simulink model "crash_original"  (R2021b)
settings: Solver=FixedStepAuto  StartTime=0.0  StopTime=10.0  RelTol=1e-3
undefined symbols (not defined in the file): DiscIntNeverNeededParam, sigbuilder_block
libraries: simulink x292, slpidlib x133
(part 1 of 12)
settings Model: Creator=cyfuzz  LastModifiedBy=cemery
settings SolverCC: AlgebraicLoopSolver=TrustRegion
settings DataIOCC: ReturnWorkspaceOutputs=off
settings DebuggingCC: SFMachineParentedDataDiag=warning  ArithmeticOperatorsInVariantConditions=warning
settings SFSimCC: SimUseLocalCustomCode=off  CustomCodeUndefinedFunction=UseInterfaceOnly
settings RTWCC: RTWUseLocalCustomCode=off
settings CodeAppCC: StateflowObjectComments=on

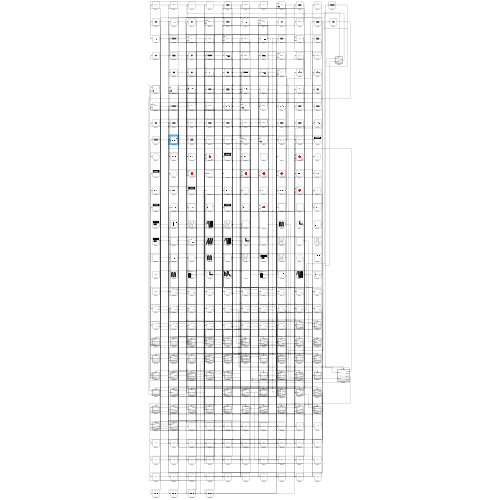
[thumbnail: Simulink's stored preview of the top-level diagram]
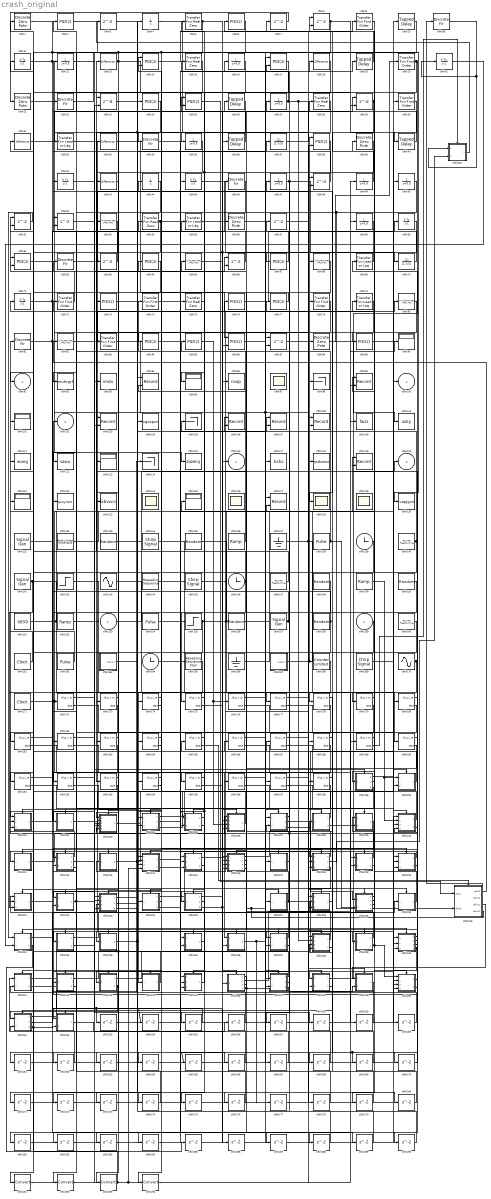
== system crash_original ==
  cfblk153 : Inport
  cfblk159 : Inport  Port=2
  cfblk{1,21,39,56,88} (5 alike) : DiscreteZeroPole  Poles=[0 0.5]  Gain=1
  cfblk{10,19,26,36,40} (5 alike) : simulink/Discrete/Tapped Delay  vinit=0.0  samptime=-1  NumDelays=1  DelayOrder=Oldest  includeCurrent=off
  cfblk{90,95,101,113,121,125} (6 alike) : Display
  cfblk103 : Record  FileSettingsInternal="{\"entries\":[{\"content\":{\"excelSettings\":{\"content\":{},\"type\":\"Streamout.ExcelSettings\"}},\"type\":\"Streamout.FileSettingStorage\",\"uuid\":\"30172691-4b6d-43b6-90c1-8d96ffbb56b2\"}],\"packageUris\":[\"http://schema.mathworks.com/mf0/streamout_blocks/R2020a\"],\"version\":\"1.0\"}"  Layout=[1 1]  SignalsInternal="{\"entries\":[{\"content\":{\"signals\":[{\"content\":{\"blockPath\":[\"crash_original/cfblk103\"],\"channel\":[],\"dimensions\":[1],\"domain\":\"crash_original/cfblk103\",\"lineColor\":\"#a2142f\",\"plots\":[1],\"port\":1,\"sid\":[],\"signalID\":25354,\"signalName\":\"XY Graph:1\"},\"type\":\"RecordBlkView.Signal\",\"uuid\":\"414546f9-114d-477c-ba68-cfa88be5a9bf\"},{\"content\":{\"blockPath\":[\"crash_original/cfblk103\"],\"channel\":[],\"dimensions\":[1],\"domain\":\"crash_original/cfblk103\",\"lineColor\":\"#139fff\",\"plots\":[1],\"port\":2,\"sid\":[],\"signalID\":25357,\"signalName\":\"XY Graph:2\"},\"type\":\"RecordBlkView.Signal\",\"uuid\":\"96b3544b-9d06-4962-b904-c7b3bf9edbf5\"}]},\"type\":\"RecordBlkView.InputSignals\",\"uuid\":\"c1b797b7-706f-480f-856e-f9fd9aac0f38\"}],\"packageUris\":[\"http://schema.mathworks.com/mf0/streamout_blocks/R2020a\"],\"version\":\"1.0\"}"  VisualizationBindings="{\"xyplotplugin\":{\"info\":[{\"series\":[{\"bindingParametersList\":[{\"parameter\":\"X-Axis\",\"signalID\":25354,\"signalName\":\"XY Graph:1\"},{\"parameter\":\"Y-Axis\",\"signalID\":25357,\"signalName\":\"XY Graph:2\"}],\"seriesID\":52165}],\"subplotID\":1}]}}"  CompatibilityTag=XY  st=-1
  cfblk104 : ToWorkspace  VariableName=cgozpzv  SaveFormat=Timeseries  SampleTime=-1
  cfblk105 : Terminator
  cfblk106 : Record  FileSettingsInternal="{\"entries\":[{\"content\":{\"excelSettings\":{\"content\":{},\"type\":\"Streamout.ExcelSettings\"}},\"type\":\"Streamout.FileSettingStorage\",\"uuid\":\"5105aa24-88b4-4d22-8fbb-db2b517dd038\"}],\"packageUris\":[\"http://schema.mathworks.com/mf0/streamout_blocks/R2020a\"],\"version\":\"1.0\"}"  Layout=[1 1]  SignalsInternal="{\"entries\":[{\"content\":{\"signals\":[{\"content\":{\"blockPath\":[\"crash_original/cfblk106\"],\"channel\":[],\"dimensions\":[1],\"domain\":\"crash_original/cfblk106\",\"lineColor\":\"#a2142f\",\"plots\":[1],\"port\":1,\"sid\":[],\"signalID\":25346,\"signalName\":\"XY Graph:1\"},\"type\":\"RecordBlkView.Signal\",\"uuid\":\"9204552f-2c26-4ac5-bb3a-39315a682c7e\"},{\"content\":{\"blockPath\":[\"crash_original/cfblk106\"],\"channel\":[],\"dimensions\":[1],\"domain\":\"crash_original/cfblk106\",\"lineColor\":\"#139fff\",\"plots\":[1],\"port\":2,\"sid\":[],\"signalID\":25349,\"signalName\":\"XY Graph:2\"},\"type\":\"RecordBlkView.Signal\",\"uuid\":\"12e95a38-9289-47da-aacf-37fae59f2bfe\"}]},\"type\":\"RecordBlkView.InputSignals\",\"uuid\":\"d2112c08-a194-4577-8bfc-846eb5e090f8\"}],\"packageUris\":[\"http://schema.mathworks.com/mf0/streamout_blocks/R2020a\"],\"version\":\"1.0\"}"  VisualizationBindings="{\"xyplotplugin\":{\"info\":[{\"series\":[{\"bindingParametersList\":[{\"parameter\":\"X-Axis\",\"signalID\":25346,\"signalName\":\"XY Graph:1\"},{\"parameter\":\"Y-Axis\",\"signalID\":25349,\"signalName\":\"XY Graph:2\"}],\"seriesID\":14933}],\"subplotID\":1}]}}"  CompatibilityTag=XY  st=-1
  cfblk107 : Record  FileSettingsInternal="{\"entries\":[{\"content\":{\"excelSettings\":{\"content\":{},\"type\":\"Streamout.ExcelSettings\"}},\"type\":\"Streamout.FileSettingStorage\",\"uuid\":\"9a455097-a817-49c6-a5c0-eb2ae5036dd7\"}],\"packageUris\":[\"http://schema.mathworks.com/mf0/streamout_blocks/R2020a\"],\"version\":\"1.0\"}"  Layout=[1 1]  SignalsInternal="{\"entries\":[{\"content\":{\"signals\":[{\"content\":{\"blockPath\":[\"crash_original/cfblk107\"],\"channel\":[],\"dimensions\":[1],\"domain\":\"crash_original/cfblk107\",\"lineColor\":\"#a2142f\",\"plots\":[1],\"port\":1,\"sid\":[],\"signalID\":25338,\"signalName\":\"XY Graph:1\"},\"type\":\"RecordBlkView.Signal\",\"uuid\":\"72b46ba4-58e1-4237-a289-6594da422004\"},{\"content\":{\"blockPath\":[\"crash_original/cfblk107\"],\"channel\":[],\"dimensions\":[1],\"domain\":\"crash_original/cfblk107\",\"lineColor\":\"#139fff\",\"plots\":[1],\"port\":2,\"sid\":[],\"signalID\":25341,\"signalName\":\"XY Graph:2\"},\"type\":\"RecordBlkView.Signal\",\"uuid\":\"e835df7f-5567-4283-ab7a-943fc1d95c97\"}]},\"type\":\"RecordBlkView.InputSignals\",\"uuid\":\"dcc1e580-6fae-4788-903d-9782004bc5fd\"}],\"packageUris\":[\"http://schema.mathworks.com/mf0/streamout_blocks/R2020a\"],\"version\":\"1.0\"}"  VisualizationBindings="{\"xyplotplugin\":{\"info\":[{\"series\":[{\"bindingParametersList\":[{\"parameter\":\"X-Axis\",\"signalID\":25338,\"signalName\":\"XY Graph:1\"},{\"parameter\":\"Y-Axis\",\"signalID\":25341,\"signalName\":\"XY Graph:2\"}],\"seriesID\":31324}],\"subplotID\":1}]}}"  CompatibilityTag=XY  st=-1
  cfblk108 : Record  FileSettingsInternal="{\"entries\":[{\"content\":{\"excelSettings\":{\"content\":{},\"type\":\"Streamout.ExcelSettings\"}},\"type\":\"Streamout.FileSettingStorage\",\"uuid\":\"0bf2bf5e-f4e3-4816-82a7-4f814904066c\"}],\"packageUris\":[\"http://schema.mathworks.com/mf0/streamout_blocks/R2020a\"],\"version\":\"1.0\"}"  Layout=[1 1]  SignalsInternal="{\"entries\":[{\"content\":{\"signals\":[{\"content\":{\"blockPath\":[\"crash_original/cfblk108\"],\"channel\":[],\"dimensions\":[1],\"domain\":\"crash_original/cfblk108\",\"lineColor\":\"#a2142f\",\"plots\":[1],\"port\":1,\"sid\":[],\"signalID\":25330,\"signalName\":\"XY Graph:1\"},\"type\":\"RecordBlkView.Signal\",\"uuid\":\"ec0f48f3-9d1b-4216-bb21-ef0bcc557efa\"},{\"content\":{\"blockPath\":[\"crash_original/cfblk108\"],\"channel\":[],\"dimensions\":[1],\"domain\":\"crash_original/cfblk108\",\"lineColor\":\"#139fff\",\"plots\":[1],\"port\":2,\"sid\":[],\"signalID\":25333,\"signalName\":\"XY Graph:2\"},\"type\":\"RecordBlkView.Signal\",\"uuid\":\"97f765a4-0795-4aab-bdad-c330e4c16f83\"}]},\"type\":\"RecordBlkView.InputSignals\",\"uuid\":\"3c2073ef-6d47-42f6-9099-379ba4442adb\"}],\"packageUris\":[\"http://schema.mathworks.com/mf0/streamout_blocks/R2020a\"],\"version\":\"1.0\"}"  VisualizationBindings="{\"xyplotplugin\":{\"info\":[{\"series\":[{\"bindingParametersList\":[{\"parameter\":\"X-Axis\",\"signalID\":25330,\"signalName\":\"XY Graph:1\"},{\"parameter\":\"Y-Axis\",\"signalID\":25333,\"signalName\":\"XY Graph:2\"}],\"seriesID\":8656}],\"subplotID\":1}]}}"  CompatibilityTag=XY  st=-1
  cfblk109 : ToFile  Filename=fwzz  SaveFormat=Timeseries
  cfblk{11,41..42,45,60,71} (6 alike) : DiscreteIntegrator  ICPrevOutput=DiscIntNeverNeededParam  ICPrevScaledInput=DiscIntNeverNeededParam
  cfblk110 : ToFile  Filename=azky  SaveFormat=Timeseries
  cfblk111 : ToFile  Filename=wang  SaveFormat=Timeseries
  cfblk112 : ToFile  Filename=sawu  SaveFormat=Timeseries
  cfblk114 : Terminator
  cfblk115 : ToWorkspace  VariableName=zazenij  SaveFormat=Timeseries  SampleTime=-1
  cfblk117 : ToFile  Filename=bshz  SaveFormat=Timeseries
  cfblk118 : ToWorkspace  VariableName=rpdzwsv  SaveFormat=Timeseries  SampleTime=-1
  cfblk119 : Record  FileSettingsInternal="{\"entries\":[{\"content\":{\"excelSettings\":{\"content\":{},\"type\":\"Streamout.ExcelSettings\"}},\"type\":\"Streamout.FileSettingStorage\",\"uuid\":\"fee27d59-1ddc-47f4-9b88-6ce813c8d426\"}],\"packageUris\":[\"http://schema.mathworks.com/mf0/streamout_blocks/R2020a\"],\"version\":\"1.0\"}"  Layout=[1 1]  SignalsInternal="{\"entries\":[{\"content\":{\"signals\":[{\"content\":{\"blockPath\":[\"crash_original/cfblk119\"],\"channel\":[],\"dimensions\":[1],\"domain\":\"crash_original/cfblk119\",\"lineColor\":\"#a2142f\",\"plots\":[1],\"port\":1,\"sid\":[],\"signalID\":25322,\"signalName\":\"XY Graph:1\"},\"type\":\"RecordBlkView.Signal\",\"uuid\":\"effbb9bf-c420-46b1-a7d1-1e032b18154d\"},{\"content\":{\"blockPath\":[\"crash_original/cfblk119\"],\"channel\":[],\"dimensions\":[1],\"domain\":\"crash_original/cfblk119\",\"lineColor\":\"#139fff\",\"plots\":[1],\"port\":2,\"sid\":[],\"signalID\":25325,\"signalName\":\"XY Graph:2\"},\"type\":\"RecordBlkView.Signal\",\"uuid\":\"bb2f82c4-e824-49d1-9fc8-a47dada03492\"}]},\"type\":\"RecordBlkView.InputSignals\",\"uuid\":\"82b3e0f0-e2fd-4ae7-a1eb-90a31382d85a\"}],\"packageUris\":[\"http://schema.mathworks.com/mf0/streamout_blocks/R2020a\"],\"version\":\"1.0\"}"  VisualizationBindings="{\"xyplotplugin\":{\"info\":[{\"series\":[{\"bindingParametersList\":[{\"parameter\":\"X-Axis\",\"signalID\":25322,\"signalName\":\"XY Graph:1\"},{\"parameter\":\"Y-Axis\",\"signalID\":25325,\"signalName\":\"XY Graph:2\"}],\"seriesID\":29524}],\"subplotID\":1}]}}"  CompatibilityTag=XY  st=-1
  cfblk{12,16,27,35,47,49..50,59} (8 alike) : DiscreteTransferFcn  SampleTime=1
  cfblk122 : ToWorkspace  VariableName=qvnyrom  SaveFormat=Timeseries  SampleTime=-1
  cfblk123 : ToWorkspace  VariableName=lxbvxco  SaveFormat=Timeseries  SampleTime=-1
  cfblk{97,124,126,128..129} (5 alike) : Scope
      cfblk124 settings: Floating=on
      cfblk126 settings: Floating=on
      cfblk129 settings: Floating=on
      cfblk97 settings: Floating=on
  cfblk127 : Record  FileSettingsInternal="{\"entries\":[{\"content\":{\"excelSettings\":{\"content\":{},\"type\":\"Streamout.ExcelSettings\"}},\"type\":\"Streamout.FileSettingStorage\",\"uuid\":\"83428cd0-c40d-4b56-9453-87c774a237f4\"}],\"packageUris\":[\"http://schema.mathworks.com/mf0/streamout_blocks/R2020a\"],\"version\":\"1.0\"}"  Layout=[1 1]  SignalsInternal="{\"entries\":[{\"content\":{\"signals\":[{\"content\":{\"blockPath\":[\"crash_original/cfblk127\"],\"channel\":[],\"dimensions\":[1],\"domain\":\"crash_original/cfblk127\",\"lineColor\":\"#a2142f\",\"plots\":[1],\"port\":1,\"sid\":[],\"signalID\":25314,\"signalName\":\"XY Graph:1\"},\"type\":\"RecordBlkView.Signal\",\"uuid\":\"4ffe00b0-219f-48e9-9eae-af36f4ef0fcf\"},{\"content\":{\"blockPath\":[\"crash_original/cfblk127\"],\"channel\":[],\"dimensions\":[1],\"domain\":\"crash_original/cfblk127\",\"lineColor\":\"#139fff\",\"plots\":[1],\"port\":2,\"sid\":[],\"signalID\":25317,\"signalName\":\"XY Graph:2\"},\"type\":\"RecordBlkView.Signal\",\"uuid\":\"f85c7929-cc6b-466a-b10c-b0d057f1a651\"}]},\"type\":\"RecordBlkView.InputSignals\",\"uuid\":\"7a008c7c-a3ea-4e7c-8ad4-a9eac3daa760\"}],\"packageUris\":[\"http://schema.mathworks.com/mf0/streamout_blocks/R2020a\"],\"version\":\"1.0\"}"  VisualizationBindings="{\"xyplotplugin\":{\"info\":[{\"series\":[{\"bindingParametersList\":[{\"parameter\":\"X-Axis\",\"signalID\":25314,\"signalName\":\"XY Graph:1\"},{\"parameter\":\"Y-Axis\",\"signalID\":25317,\"signalName\":\"XY Graph:2\"}],\"seriesID\":431}],\"subplotID\":1}]}}"  CompatibilityTag=XY  st=-1
  cfblk{13,18,31,33,43} (5 alike) : simulink/Discrete/Difference  ICPrevInput=0.0  OutMin=[]  OutMax=[]  OutDataTypeStr=Inherit: Inherit via back propagation  OutDataType=fixdt(1, 16)  OutScaling=2^-10  DoSatur=off
  cfblk130 : ToWorkspace  VariableName=vapjgvn  SaveFormat=Timeseries  SampleTime=-1
  cfblk131 : SignalGenerator  Units=rad/sec
  cfblk132 : simulink/Sources/Band-Limited White Noise  Cov=[0.1]  Ts=0.1  seed=[23341]
  cfblk{133,135,148,156,158} (5 alike) : UniformRandomNumber  SampleTime=0.1
  cfblk134 : simulink/Sources/Chirp Signal  f1=0.1  T=100  f2=1
  cfblk136 : simulink/Sources/Ramp  slope=1  start=0  InitialOutput=0
  cfblk137 : Ground
  cfblk138 : DiscretePulseGenerator  PulseType=Time based  Period=10  PulseWidth=5
  cfblk139 : Clock
  cfblk{14,17,25,38,61,86} (6 alike) : slpidlib/PID Controller (2DOF)  Controller=PID  Form=Parallel  TimeDomain=Discrete-time  UseExternalTs=off  SampleTime=1  IntegratorMethod=Forward Euler  FilterMethod=Forward Euler  ControllerParametersSource=internal  P=1  I=1  D=0  UseFilter=on  N=100  b=1  c=1  TunerSelectOption=Transfer Function Based (PID Tuner App)  InitialConditionSource=internal  InitialConditionForIntegrator=0  InitialConditionForFilter=0  DifferentiatorICPrevScaledInput=0  ExternalReset=none  TrackingMode=off  Kt=1  LimitOutput=off  SatLimitsSource=internal  UpperSaturationLimit=inf  LowerSaturationLimit=-inf  LinearizeAsGain=off  AntiWindupMode=none  Kb=1  POutMin=[]  POutMax=[]  IOutMin=[]  IOutMax=[]  DOutMin=[]  DOutMax=[]  NOutMin=[]  NOutMax=[]  bOutMin=[]  bOutMax=[]  cOutMin=[]  cOutMax=[]  SumOutMin=[]  SumOutMax=[]  SaturationOutMin=[]  SaturationOutMax=[]  PParamMin=[]  PParamMax=[]  IParamMin=[]  IParamMax=[]  DParamMin=[]  DParamMax=[]  NParamMin=[]  NParamMax=[]  bParamMin=[]  bParamMax=[]  cParamMin=[]  cParamMax=[]  KbParamMin=[]  KbParamMax=[]  KtParamMin=[]  KtParamMax=[]  KbOutMin=[]  KbOutMax=[]  KtOutMin=[]  KtOutMax=[]  IntegratorOutMin=[]  IntegratorOutMax=[]  FilterOutMin=[]  FilterOutMax=[]  SumI1OutMin=[]  SumI1OutMax=[]  SumI2OutMin=[]  SumI2OutMax=[]  SumI3OutMin=[]  SumI3OutMax=[]  SumI4OutMin=[]  SumI4OutMax=[]  SumDOutMin=[]  SumDOutMax=[]  Sum1OutMin=[]  Sum1OutMax=[]  Sum2OutMin=[]  Sum2OutMax=[]  Sum3OutMin=[]  Sum3OutMax=[]  DifferentiatorOutMin=[]  DifferentiatorOutMax=[]  FilterDiffOutCoefMin=[]  FilterDiffOutCoefMax=[]  ReciprocalOutMin=[]  ReciprocalOutMax=[]  SumDenOutMin=[]  SumDenOutMax=[]  SumNumOutMin=[]  SumNumOutMax=[]  DivideOutMin=[]  DivideOutMax=[]  UdiffTsProdOutMin=[]  UdiffTsProdOutMax=[]  NTsProdOutMin=[]  NTsProdOutMax=[]  UintegralTsProdOutMin=[]  UintegralTsProdOutMax=[]  UngainTsProdOutMin=[]  UngainTsProdOutMax=[]  IntegratorContinuousStateAttributes=''  IntegratorStateMustResolveToSignalObject=off  IntegratorRTWStateStorageClass=Auto  FilterContinuousStateAttributes=''  FilterStateMustResolveToSignalObject=off  FilterRTWStateStorageClass=Auto  ParallelPVariant=InternalParameters  IdealPVariant=Disabled  IVariant=InternalParameters  DVariant=InternalParameters  bVariant=InternalParameters  cVariant=InternalParameters  IntegratorVariant=Discrete  SatVariant=Disabled  AWVariant=Passthrough  PCopyVariant=Disabled  TRVariant=Disabled  FdbkBlocksVariant=Forward  IdealPFdbkVariant=Disabled  SatFdbkVariant=Disabled  DerivativeFilterVariant=ForwardEulerFilter  NVariant=InternalParameters  NCopyVariant=Disabled  FilterICVariant=InternalICsFilter  IntegratorICVariant=InternalICs  ExternalResetVariant=Disabled  TRSumVariant=Passthrough  SumFdbkVariant=Disabled  SumVariant=Sum_PID  TsampFilterVariant=InternalTs  TsampNgainVariant=Passthrough  TsampIntegralVariant=Passthrough  ExternalSaturationOutDataTypeStr=Inherit: Same as second input
      settings: SourceProductBaseCode=SL
  cfblk140 : simulink/Sources/Counter Free-Running  NumBits=16  tsamp=-1
  cfblk141 : SignalGenerator  Units=rad/sec
  cfblk142 : Step  After=57  SampleTime=0
  cfblk143 : Sin  SampleTime=0
  cfblk144 : simulink/Sources/Repeating Sequence  rep_seq_t=[0 2]  rep_seq_y=[0 2]
  cfblk145 : simulink/Sources/Chirp Signal  f1=0.1  T=100  f2=1
  cfblk146 : Clock
  cfblk147 : simulink/Sources/Counter Free-Running  NumBits=16  tsamp=-1
  cfblk149 : simulink/Sources/Ramp  slope=1  start=0  InitialOutput=0
  cfblk{5,15,28,54,75} (5 alike) : simulink/Discrete/Transfer Fcn Real Zero  ZeroZ=0.75  ICPrevInput=0.0  DoSatur=off
      settings: SourceProductBaseCode=SL
  cfblk150 : RandomNumber  SampleTime=0.1
  cfblk151 : Constant  Value=9859
  cfblk152 : simulink/Sources/Ramp  slope=1  start=0  InitialOutput=0
  cfblk154 : DiscretePulseGenerator  PulseType=Time based  Period=10  PulseWidth=5
  cfblk155 : Step  After=75  SampleTime=0
  cfblk157 : SignalGenerator  Units=rad/sec
  cfblk160 : simulink/Sources/Counter Free-Running  NumBits=16  tsamp=-1
  cfblk161 : DigitalClock
  cfblk162 : DiscretePulseGenerator  PulseType=Time based  Period=10  PulseWidth=5
  cfblk163 : Subsystem  Tag=STV Subsys  LoadFcn=sigbuilder_block('load');  StartFcn=sigbuilder_block('start');  StopFcn=sigbuilder_block('stop');  ClipboardFcn=sigbuilder_block('clipboard');  mask(Sigbuilder block){tuvar=[0:10]}
      mask help: Simulink:masks:SigbuilderBlock_MD
      mask init:
      | if ~strcmp(get_param(bdroot(gcbh),'SimulationStatus'),'stopped') tuvar = sigbuilder_block('maskInit'); end
      settings: CopyFcn=sigbuilder_block('copy');  DeleteFcn=sigbuilder_block('delete');  ModelCloseFcn=sigbuilder_block('modelClose');  PreSaveFcn=sigbuilder_block('preSave');  PauseFcn=sigbuilder_block('pause');  ContinueFcn=sigbuilder_block('continue');  NameChangeFcn=sigbuilder_block('namechange');  OpenFcn=sigbuilder_block('open',[437.6 199.2 550.4 400 ]);  CloseFcn=sigbuilder_block('close');
      mask Display: plot(0, 0, 100, 100,[2, 2, 32, 32, 2], [68, 8, 8, 68, 68],[32, 2], [38, 38], [32, 19, 2],[53, 60, 44], [32, 17, 17, 2],[16, 16, 31, 31]);txt = getActiveGroup(gcbh);text(2, 100, txt,'verticalAlignment', 'top');
  cfblk164 : Clock
  cfblk165 : simulink/Sources/Repeating Sequence Stair  OutValues=[3 1 4 2 1].'  tsamp=-1  OutMin=[]  OutMax=[]  OutDataTypeStr=double  OutputDataTypeScalingMode=double  OutDataType=fixdt(0,8)  ConRadixGroup=Best Precision: Vector-wise  OutScaling=2^-12
  cfblk166 : Ground
  cfblk167 : Subsystem  Tag=STV Subsys  LoadFcn=sigbuilder_block('load');  StartFcn=sigbuilder_block('start');  StopFcn=sigbuilder_block('stop');  ClipboardFcn=sigbuilder_block('clipboard');  mask(Sigbuilder block){tuvar=[0:10]}
      mask help: Simulink:masks:SigbuilderBlock_MD
      mask init:
      | if ~strcmp(get_param(bdroot(gcbh),'SimulationStatus'),'stopped') tuvar = sigbuilder_block('maskInit'); end
      settings: CopyFcn=sigbuilder_block('copy');  DeleteFcn=sigbuilder_block('delete');  ModelCloseFcn=sigbuilder_block('modelClose');  PreSaveFcn=sigbuilder_block('preSave');  PauseFcn=sigbuilder_block('pause');  ContinueFcn=sigbuilder_block('continue');  NameChangeFcn=sigbuilder_block('namechange');  OpenFcn=sigbuilder_block('open',[437.6 199.2 550.4 400 ]);  CloseFcn=sigbuilder_block('close');
      mask Display: plot(0, 0, 100, 100,[2, 2, 32, 32, 2], [68, 8, 8, 68, 68],[32, 2], [38, 38], [32, 19, 2],[53, 60, 44], [32, 17, 17, 2],[16, 16, 31, 31]);txt = getActiveGroup(gcbh);text(2, 100, txt,'verticalAlignment', 'top');
  cfblk168 : simulink/Sources/Counter Limited  uplimit=7  tsamp=-1
  cfblk169 : simulink/Sources/Chirp Signal  f1=0.1  T=100  f2=1
  cfblk170 : Sin  SampleTime=0
  cfblk171 : DigitalClock
  cfblk{172..198} (27 alike) : If  SampleTime=1
  cfblk199 : Subsystem  TreatAsAtomicUnit=on
  cfblk{2,6,24,64,67,73,76..77,84..85,89} (11 alike) : slpidlib/PID Controller  Controller=PID  Form=Parallel  TimeDomain=Discrete-time  UseExternalTs=off  SampleTime=1  IntegratorMethod=Forward Euler  FilterMethod=Forward Euler  ControllerParametersSource=internal  P=1  I=1  D=0  UseFilter=on  N=100  TunerSelectOption=Transfer Function Based (PID Tuner App)  InitialConditionSource=internal  InitialConditionForIntegrator=0  InitialConditionForFilter=0  DifferentiatorICPrevScaledInput=0  ExternalReset=none  TrackingMode=off  Kt=1  LimitOutput=off  SatLimitsSource=internal  UpperSaturationLimit=inf  LowerSaturationLimit=-inf  LinearizeAsGain=off  AntiWindupMode=none  Kb=1  POutMin=[]  POutMax=[]  IOutMin=[]  IOutMax=[]  DOutMin=[]  DOutMax=[]  NOutMin=[]  NOutMax=[]  SumOutMin=[]  SumOutMax=[]  SaturationOutMin=[]  SaturationOutMax=[]  PParamMin=[]  PParamMax=[]  IParamMin=[]  IParamMax=[]  DParamMin=[]  DParamMax=[]  NParamMin=[]  NParamMax=[]  KbParamMin=[]  KbParamMax=[]  KtParamMin=[]  KtParamMax=[]  KbOutMin=[]  KbOutMax=[]  KtOutMin=[]  KtOutMax=[]  IntegratorOutMin=[]  IntegratorOutMax=[]  FilterOutMin=[]  FilterOutMax=[]  SumI1OutMin=[]  SumI1OutMax=[]  SumI2OutMin=[]  SumI2OutMax=[]  SumI3OutMin=[]  SumI3OutMax=[]  SumI4OutMin=[]  SumI4OutMax=[]  SumDOutMin=[]  SumDOutMax=[]  DifferentiatorOutMin=[]  DifferentiatorOutMax=[]  FilterDiffOutCoefMin=[]  FilterDiffOutCoefMax=[]  ReciprocalOutMin=[]  ReciprocalOutMax=[]  SumDenOutMin=[]  SumDenOutMax=[]  SumNumOutMin=[]  SumNumOutMax=[]  DivideOutMin=[]  DivideOutMax=[]  UdiffTsProdOutMin=[]  UdiffTsProdOutMax=[]  NTsProdOutMin=[]  NTsProdOutMax=[]  UintegralTsProdOutMin=[]  UintegralTsProdOutMax=[]  UngainTsProdOutMin=[]  UngainTsProdOutMax=[]  IntegratorContinuousStateAttributes=''  IntegratorStateMustResolveToSignalObject=off  IntegratorRTWStateStorageClass=Auto  FilterContinuousStateAttributes=''  FilterStateMustResolveToSignalObject=off  FilterRTWStateStorageClass=Auto  ParallelPVariant=InternalParameters  IdealPVariant=Disabled  IVariant=InternalParameters  DVariant=InternalParameters  IntegratorVariant=Discrete  SatVariant=Disabled  AWVariant=Passthrough  PCopyVariant=Disabled  TRVariant=Disabled  FdbkBlocksVariant=Forward  IdealPFdbkVariant=Disabled  SatFdbkVariant=Disabled  DerivativeFilterVariant=ForwardEulerFilter  NVariant=InternalParameters  NCopyVariant=Disabled  FilterICVariant=InternalICsFilter  IntegratorICVariant=InternalICs  ExternalResetVariant=Disabled  TRSumVariant=Passthrough  SumFdbkVariant=Disabled  SumVariant=Sum_PID  TsampFilterVariant=InternalTs  TsampNgainVariant=Passthrough  TsampIntegralVariant=Passthrough  ExternalSaturationOutDataTypeStr=Inherit: Same as second input
  cfblk{9,20,30,72,74,78,83} (7 alike) : simulink/Discrete/Transfer Fcn First Order  PoleZ=0.95  ICPrevOutput=0.0  DoSatur=off
  cfblk200 : Subsystem  TreatAsAtomicUnit=on
  cfblk201 : Subsystem  TreatAsAtomicUnit=on
  cfblk202 : Subsystem  TreatAsAtomicUnit=on
  cfblk203 : Subsystem  TreatAsAtomicUnit=on
  cfblk204 : Subsystem  TreatAsAtomicUnit=on
  cfblk205 : Subsystem  TreatAsAtomicUnit=on
  cfblk206 : Subsystem  TreatAsAtomicUnit=on
  cfblk207 : Subsystem  TreatAsAtomicUnit=on
  cfblk208 : Subsystem  TreatAsAtomicUnit=on
  cfblk209 : Subsystem  TreatAsAtomicUnit=on
  cfblk210 : Subsystem  TreatAsAtomicUnit=on
  cfblk211 : Subsystem  TreatAsAtomicUnit=on
  cfblk212 : Subsystem  TreatAsAtomicUnit=on
  cfblk213 : Subsystem  TreatAsAtomicUnit=on
  cfblk214 : Subsystem  TreatAsAtomicUnit=on
  cfblk215 : Subsystem  TreatAsAtomicUnit=on
  cfblk216 : Subsystem  TreatAsAtomicUnit=on
  cfblk217 : Subsystem  TreatAsAtomicUnit=on
  cfblk218 : Subsystem  TreatAsAtomicUnit=on
  cfblk219 : Subsystem  TreatAsAtomicUnit=on
  cfblk{22,34,46,58,62,81} (6 alike) : DiscreteFir  SampleTime=1
  cfblk220 : Subsystem  TreatAsAtomicUnit=on
  cfblk221 : Subsystem  TreatAsAtomicUnit=on
  cfblk222 : Subsystem  TreatAsAtomicUnit=on
  cfblk223 : Subsystem  TreatAsAtomicUnit=on
  cfblk224 : Subsystem  TreatAsAtomicUnit=on
  cfblk225 : Subsystem  TreatAsAtomicUnit=on
  cfblk226 : Subsystem  TreatAsAtomicUnit=on
  cfblk227 : Subsystem  TreatAsAtomicUnit=on
  cfblk228 : Subsystem  TreatAsAtomicUnit=on
  cfblk229 : Subsystem  TreatAsAtomicUnit=on
  cfblk23 : Delay  DelayLengthSource=Input port  SampleTime=1
      settings: InputPortMap=u0,p1
  cfblk230 : Subsystem  TreatAsAtomicUnit=on
  cfblk231 : Subsystem  TreatAsAtomicUnit=on
  cfblk232 : Subsystem  TreatAsAtomicUnit=on
  cfblk233 : Subsystem  TreatAsAtomicUnit=on
  cfblk234 : Subsystem  TreatAsAtomicUnit=on
  cfblk235 : Subsystem  TreatAsAtomicUnit=on
  cfblk236 : Subsystem  TreatAsAtomicUnit=on
  cfblk237 : Subsystem  TreatAsAtomicUnit=on
  cfblk238 : Subsystem  TreatAsAtomicUnit=on
  cfblk239 : Subsystem  TreatAsAtomicUnit=on
  cfblk240 : Subsystem  TreatAsAtomicUnit=on
  cfblk241 : Subsystem  TreatAsAtomicUnit=on
  cfblk242 : Subsystem  TreatAsAtomicUnit=on
  cfblk243 : Subsystem  TreatAsAtomicUnit=on
  cfblk244 : Subsystem  TreatAsAtomicUnit=on
  cfblk245 : Subsystem  TreatAsAtomicUnit=on
  cfblk246 : Subsystem  TreatAsAtomicUnit=on
  cfblk247 : Subsystem  TreatAsAtomicUnit=on
  cfblk248 : Subsystem  TreatAsAtomicUnit=on
  cfblk249 : Subsystem  TreatAsAtomicUnit=on
  cfblk250 : Subsystem  TreatAsAtomicUnit=on
  cfblk251 : Subsystem  TreatAsAtomicUnit=on
  cfblk252 : Subsystem  TreatAsAtomicUnit=on
  cfblk{3,7,57,63,253..290} (42 alike) : Delay  SampleTime=1
  cfblk29 : Delay  DelayLengthSource=Input port  SampleTime=1
      settings: InputPortMap=u0,p1
  cfblk{291..294} (4 alike) : DataTypeConversion
  cfblk{32,55,69,79} (4 alike) : simulink/Discrete/Transfer Fcn Lead or Lag  PoleZ=0.95  ZeroZ=0.75  ICPrevOutput=0.0  ICPrevInput=0.0  DoSatur=off
      settings: SourceProductBaseCode=SL
  cfblk37 : DiscreteFilter  SampleTime=1
  cfblk4 : UnitDelay  HasFrameUpgradeWarning=on
  cfblk44 : UnitDelay  HasFrameUpgradeWarning=on
  cfblk48 : Delay  DelayLengthSource=Input port  SampleTime=1
      settings: InputPortMap=u0,p1
  cfblk{8,51..52,66,87} (5 alike) : Delay  ShowEnablePort=on  SampleTime=1
      settings: InputPortMap=u0,e6
  cfblk{53,65,68,80,82} (5 alike) : DiscreteStateSpace
  cfblk70 : DiscreteFilter  SampleTime=1
  cfblk92 : ToWorkspace  VariableName=muhrgrf  SaveFormat=Timeseries  SampleTime=-1
  cfblk93 : ToFile  Filename=imdo  SaveFormat=Timeseries
  cfblk94 : Record  FileSettingsInternal="{\"entries\":[{\"content\":{\"excelSettings\":{\"content\":{},\"type\":\"Streamout.ExcelSettings\"}},\"type\":\"Streamout.FileSettingStorage\",\"uuid\":\"b24fa2aa-e125-405a-9ac1-a38bed6d1bae\"}],\"packageUris\":[\"http://schema.mathworks.com/mf0/streamout_blocks/R2020a\"],\"version\":\"1.0\"}"  Layout=[1 1]  SignalsInternal="{\"entries\":[{\"content\":{\"signals\":[{\"content\":{\"blockPath\":[\"crash_original/cfblk94\"],\"channel\":[],\"dimensions\":[1],\"domain\":\"crash_original/cfblk94\",\"lineColor\":\"#a2142f\",\"plots\":[1],\"port\":1,\"sid\":[],\"signalID\":25306,\"signalName\":\"XY Graph:1\"},\"type\":\"RecordBlkView.Signal\",\"uuid\":\"67cb8b8d-4651-489b-a766-61326855b940\"},{\"content\":{\"blockPath\":[\"crash_original/cfblk94\"],\"channel\":[],\"dimensions\":[1],\"domain\":\"crash_original/cfblk94\",\"lineColor\":\"#139fff\",\"plots\":[1],\"port\":2,\"sid\":[],\"signalID\":25309,\"signalName\":\"XY Graph:2\"},\"type\":\"RecordBlkView.Signal\",\"uuid\":\"ecb52028-bf62-4b2d-82ed-da68aeeccf4b\"}]},\"type\":\"RecordBlkView.InputSignals\",\"uuid\":\"0fec34b7-277f-4bb8-a879-22d04ef37f00\"}],\"packageUris\":[\"http://schema.mathworks.com/mf0/streamout_blocks/R2020a\"],\"version\":\"1.0\"}"  VisualizationBindings="{\"xyplotplugin\":{\"info\":[{\"series\":[{\"bindingParametersList\":[{\"parameter\":\"X-Axis\",\"signalID\":25306,\"signalName\":\"XY Graph:1\"},{\"parameter\":\"Y-Axis\",\"signalID\":25309,\"signalName\":\"XY Graph:2\"}],\"seriesID\":39593}],\"subplotID\":1}]}}"  CompatibilityTag=XY  st=-1
  cfblk96 : ToFile  Filename=nvap  SaveFormat=Timeseries
  cfblk98 : Terminator
  cfblk99 : Record  FileSettingsInternal="{\"entries\":[{\"content\":{\"excelSettings\":{\"content\":{},\"type\":\"Streamout.ExcelSettings\"}},\"type\":\"Streamout.FileSettingStorage\",\"uuid\":\"5049ec40-0b2c-47bf-94c0-93020c87f72b\"}],\"packageUris\":[\"http://schema.mathworks.com/mf0/streamout_blocks/R2020a\"],\"version\":\"1.0\"}"  Layout=[1 1]  SignalsInternal="{\"entries\":[{\"content\":{\"signals\":[{\"content\":{\"blockPath\":[\"crash_original/cfblk99\"],\"channel\":[],\"dimensions\":[1],\"domain\":\"crash_original/cfblk99\",\"lineColor\":\"#a2142f\",\"plots\":[1],\"port\":1,\"sid\":[],\"signalID\":25298,\"signalName\":\"XY Graph:1\"},\"type\":\"RecordBlkView.Signal\",\"uuid\":\"94debffc-6a56-4031-bc1f-807cd091ef66\"},{\"content\":{\"blockPath\":[\"crash_original/cfblk99\"],\"channel\":[],\"dimensions\":[1],\"domain\":\"crash_original/cfblk99\",\"lineColor\":\"#139fff\",\"plots\":[1],\"port\":2,\"sid\":[],\"signalID\":25301,\"signalName\":\"XY Graph:2\"},\"type\":\"RecordBlkView.Signal\",\"uuid\":\"ec180e15-ea40-45ae-b280-3fc0ed718c5d\"}]},\"type\":\"RecordBlkView.InputSignals\",\"uuid\":\"6ad28fd7-5642-426a-8ace-02cf3ea0d04a\"}],\"packageUris\":[\"http://schema.mathworks.com/mf0/streamout_blocks/R2020a\"],\"version\":\"1.0\"}"  VisualizationBindings="{\"xyplotplugin\":{\"info\":[{\"series\":[{\"bindingParametersList\":[{\"parameter\":\"X-Axis\",\"signalID\":25298,\"signalName\":\"XY Graph:1\"},{\"parameter\":\"Y-Axis\",\"signalID\":25301,\"signalName\":\"XY Graph:2\"}],\"seriesID\":65304}],\"subplotID\":1}]}}"  CompatibilityTag=XY  st=-1
  cfblk91 : Outport  VectorParamsAs1DForOutWhenUnconnected=off
  cfblk100 : Outport  Port=2  VectorParamsAs1DForOutWhenUnconnected=off
  cfblk102 : Outport  Port=3  VectorParamsAs1DForOutWhenUnconnected=off
  cfblk116 : Outport  Port=4  VectorParamsAs1DForOutWhenUnconnected=off
  cfblk120 : Outport  Port=5  VectorParamsAs1DForOutWhenUnconnected=off
  wires:
  cfblk224/1(cfblk2) -> cfblk80/1
  cfblk168/1 -> cfblk178/1
  cfblk21/1 -> cfblk35/1
  cfblk85/1 -> cfblk176/1, cfblk206/3(cfblk15)
  cfblk165/1 -> cfblk244/1(cfblk1)
  cfblk249/1(cfblk2) -> cfblk114/1
  cfblk207/1(cfblk2) -> cfblk243/1(cfblk1)
  cfblk248/1(cfblk2) -> cfblk69/1
  cfblk81/1 -> cfblk115/1, cfblk203/3(cfblk14)
  cfblk156/1 -> cfblk50/1
  cfblk76/1 -> cfblk60/1
  cfblk138/1 -> cfblk74/1, cfblk229/2(cfblk11)
  cfblk149/1 -> cfblk200/1(cfblk1), cfblk210/2(cfblk9)
  cfblk147/1 -> cfblk13/1
  cfblk22/1 -> cfblk130/1
  cfblk3/1 -> cfblk224/1(cfblk1)
  cfblk32/1 -> cfblk239/1(cfblk1)
  cfblk161/1 -> cfblk81/1
  cfblk240/1(cfblk2) -> cfblk102/1
  cfblk20/1 -> cfblk91/1, cfblk290/1
  cfblk4/1 -> cfblk188/1
  cfblk239/1(cfblk2) -> cfblk66/1
  cfblk217/1(cfblk2) -> cfblk47/1
  cfblk53/1 -> cfblk192/1
  cfblk170/1 -> cfblk120/1, cfblk221/2(cfblk14)
  cfblk157/1 -> cfblk122/1, cfblk237/1(cfblk1)
  cfblk47/1 -> cfblk70/1, cfblk257/1
  cfblk24/1 -> cfblk193/1
  cfblk135/1 -> cfblk179/1
  cfblk167/1(Signal 1) -> cfblk38/1, cfblk119/2
  cfblk158/1 -> cfblk77/1, cfblk204/1(cfblk1)
  cfblk133/1 -> cfblk36/1
  cfblk218/1(cfblk2) -> cfblk55/1
  cfblk207/2(cfblk14) -> cfblk229/1(cfblk1)
  cfblk13/1 -> cfblk233/1(cfblk1), cfblk127/1
  cfblk132/1 -> cfblk104/1
  cfblk39/1 -> cfblk103/1
  cfblk142/1 -> cfblk200/2(cfblk8)
  cfblk229/1(cfblk2) -> cfblk232/1(cfblk1)
  cfblk37/1 -> cfblk9/1
  cfblk171/1 -> cfblk236/1(cfblk1), cfblk23/2
  cfblk29/1 -> cfblk128/1, cfblk279/1
  cfblk35/1 -> cfblk194/1
  cfblk247/1(cfblk2) -> cfblk182/1
  cfblk203/1(cfblk2) -> cfblk116/1
  cfblk243/1(cfblk2) -> cfblk109/1
  cfblk9/1 -> cfblk199/1(cfblk1)
  cfblk238/1(cfblk2) -> cfblk57/1
  cfblk235/1(cfblk2) -> cfblk5/1
  cfblk215/1(cfblk2) -> cfblk98/1
  cfblk222/1(cfblk2) -> cfblk33/1, cfblk172/1
  cfblk144/1 -> cfblk190/1
  cfblk248/2(cfblk9) -> cfblk43/1
  cfblk31/1 -> cfblk27/1
  cfblk72/1 -> cfblk51/1
  cfblk11/1 -> cfblk197/1, cfblk25/2
  cfblk145/1 -> cfblk227/1(cfblk1)
  cfblk63/1 -> cfblk12/1
  cfblk33/1 -> cfblk86/1
  cfblk49/1 -> cfblk8/1
  cfblk152/1 -> cfblk174/1
  cfblk89/1 -> cfblk30/1
  cfblk232/1(cfblk2) -> cfblk86/2
  cfblk238/2(cfblk9) -> cfblk42/1
  cfblk216/1(cfblk2) -> cfblk48/1
  cfblk36/1 -> cfblk2/1
  cfblk58/1 -> cfblk234/1(cfblk1), cfblk41/1
  cfblk246/2(cfblk12) -> cfblk90/1
  cfblk204/1(cfblk2) -> cfblk10/1
  cfblk241/1(cfblk2) -> cfblk180/1
  cfblk151/1 -> cfblk207/1(cfblk1), cfblk99/2
  cfblk230/1(cfblk2) -> cfblk39/1
  cfblk28/1 -> cfblk123/1, cfblk204/2(cfblk11)
  cfblk42/1 -> cfblk29/1
  cfblk83/1 -> cfblk235/1(cfblk1)
  cfblk159/1 -> cfblk183/1
  cfblk45/1 -> cfblk228/1(cfblk1)
  cfblk87/1 -> cfblk20/1
  cfblk88/1 -> cfblk110/1
  cfblk242/1(cfblk2) -> cfblk118/1
  cfblk218/2(cfblk15) -> cfblk234/2(cfblk15)
  cfblk16/1 -> cfblk195/1
  cfblk6/1 -> cfblk272/1, cfblk273/1, cfblk274/1
  cfblk27/1 -> cfblk238/2(cfblk6), cfblk250/3(cfblk13), cfblk15/1
  cfblk66/1 -> cfblk46/1
  cfblk75/1 -> cfblk225/1(cfblk1)
  cfblk68/1 -> cfblk196/1
  cfblk202/1(cfblk2) -> cfblk45/1
  cfblk207/3(cfblk15) -> cfblk49/1
  cfblk244/1(cfblk2) -> cfblk51/2, cfblk223/3(cfblk11)
  cfblk12/1 -> cfblk29/2
  cfblk245/1(cfblk2) -> cfblk85/1
  cfblk62/1 -> cfblk38/2
  cfblk139/1 -> cfblk202/1(cfblk1)
  cfblk77/1 -> cfblk73/1
  cfblk212/1(cfblk2) -> cfblk101/1
  cfblk82/1 -> cfblk17/1
  cfblk251/1(cfblk2) -> cfblk24/1
  cfblk219/1(cfblk2) -> cfblk209/1(cfblk1)
  cfblk213/1(cfblk2) -> cfblk75/1, cfblk250/4(cfblk14)
  cfblk153/1 -> cfblk100/1
  cfblk227/1(cfblk2) -> cfblk230/1(cfblk1), cfblk203/5(cfblk16)
  cfblk5/1 -> cfblk107/2, cfblk108/2, cfblk181/1
  cfblk10/1 -> cfblk34/1
  cfblk69/1 -> cfblk67/1
  cfblk19/1 -> cfblk6/1
  cfblk25/1 -> cfblk226/1(cfblk1)
  cfblk43/1 -> cfblk173/1
  cfblk14/1 -> cfblk8/2
  cfblk70/1 -> cfblk17/2
  cfblk7/1 -> cfblk21/1
  cfblk140/1 -> cfblk211/1(cfblk1), cfblk106/2
  cfblk206/1(cfblk2) -> cfblk121/1
  cfblk226/1(cfblk2) -> cfblk82/1
  cfblk160/1 -> cfblk191/1
  cfblk64/1 -> cfblk201/1(cfblk1)
  cfblk78/1 -> cfblk293/1
  cfblk216/2(cfblk13) -> cfblk113/1
  cfblk67/1 -> cfblk54/1
  cfblk205/1(cfblk2) -> cfblk222/1(cfblk1)
  cfblk2/1 -> cfblk87/2
  cfblk131/1 -> cfblk222/2(cfblk17)
  cfblk237/1(cfblk2) -> cfblk63/1
  cfblk17/1 -> cfblk223/2(cfblk10)
  cfblk154/1 -> cfblk219/1(cfblk1)
  cfblk71/1 -> cfblk108/1, cfblk223/4(cfblk12)
  cfblk86/1 -> cfblk79/1
  cfblk26/1 -> cfblk203/1(cfblk1)
  cfblk211/1(cfblk2) -> cfblk206/1(cfblk1)
  cfblk234/1(cfblk2) -> cfblk3/1
  cfblk224/3(cfblk13) -> cfblk19/1
  cfblk54/1 -> cfblk103/2, cfblk266/1
  cfblk1/1 -> cfblk247/2(cfblk15), cfblk14/2
  cfblk79/1 -> cfblk235/2(cfblk7)
  cfblk61/1 -> cfblk253/1, cfblk254/1
  cfblk55/1 -> cfblk117/1
  cfblk200/1(cfblk2) -> cfblk111/1
  cfblk8/1 -> cfblk40/1, cfblk203/4(cfblk15)
  cfblk247/2(cfblk16) -> cfblk185/1
  cfblk214/1(cfblk2) -> cfblk16/1
  cfblk80/1 -> cfblk89/1
  cfblk247/3(cfblk17) -> cfblk241/2(cfblk9)
  cfblk236/1(cfblk2) -> cfblk238/3(cfblk7), cfblk277/1
  cfblk223/1(cfblk2) -> cfblk94/1
  cfblk212/3(cfblk17) -> cfblk62/1
  cfblk239/2(cfblk7) -> cfblk221/1(cfblk1), cfblk250/1(cfblk1)
  cfblk48/1 -> cfblk23/1
  cfblk148/1 -> cfblk206/2(cfblk14)
  cfblk40/1 -> cfblk26/1
  cfblk166/1 -> cfblk68/1
  cfblk225/1(cfblk2) -> cfblk236/2(cfblk8)
  cfblk225/2(cfblk14) -> cfblk53/1
  cfblk51/1 -> cfblk231/1(cfblk1)
  cfblk143/1 -> cfblk245/2(cfblk12)
  cfblk134/1 -> cfblk177/1
  cfblk18/1 -> cfblk95/1
  cfblk65/1 -> cfblk28/1
  cfblk50/1 -> cfblk205/2(cfblk9), cfblk226/2(cfblk9)
  cfblk216/3(cfblk14) -> cfblk44/1
  cfblk246/3(cfblk13) -> cfblk94/2
  cfblk242/2(cfblk10) -> cfblk52/1
  cfblk226/2(cfblk10) -> cfblk58/1
  cfblk169/1 -> cfblk240/1(cfblk1)
  cfblk30/1 -> cfblk240/2(cfblk13)
  cfblk226/3(cfblk11) -> cfblk249/1(cfblk1)
  cfblk215/2(cfblk15) -> cfblk61/1
  cfblk137/1 -> cfblk238/1(cfblk1), cfblk250/2(cfblk12)
  cfblk232/2(cfblk11) -> cfblk65/1
  cfblk243/2(cfblk17) -> cfblk251/1(cfblk1), cfblk22/1
  cfblk251/2(cfblk9) -> cfblk228/2(cfblk14)
  cfblk208/1(cfblk2) -> cfblk14/1
  cfblk226/4(cfblk12) -> cfblk105/1, cfblk18/1
  cfblk219/2(cfblk11) -> cfblk99/1
  cfblk38/1 -> cfblk205/1(cfblk1), cfblk275/1, cfblk83/1
  cfblk41/1 -> cfblk231/2(cfblk14)
  cfblk162/1 -> cfblk61/2
  cfblk136/1 -> cfblk52/2
  cfblk233/1(cfblk2) -> cfblk37/1, cfblk258/1
  cfblk163/1(Signal 1) -> cfblk4/1
  cfblk201/1(cfblk2) -> cfblk56/1
  cfblk73/1 -> cfblk240/3(cfblk14)
  cfblk210/1(cfblk2) -> cfblk64/1
  cfblk15/1 -> cfblk84/1
  cfblk74/1 -> cfblk248/1(cfblk1)
  cfblk141/1 -> cfblk245/3(cfblk13), cfblk221/3(cfblk15)
  cfblk60/1 -> cfblk112/1, cfblk206/4(cfblk16)
  cfblk146/1 -> cfblk175/1, cfblk31/1
  cfblk216/4(cfblk15) -> cfblk72/1
  cfblk155/1 -> cfblk228/3(cfblk15), cfblk127/2, cfblk214/2(cfblk12)
  cfblk251/3(cfblk10) -> cfblk201/2(cfblk12), cfblk287/1
  cfblk214/2(cfblk15) -> cfblk218/1(cfblk1)
  cfblk237/2(cfblk7) -> cfblk203/2(cfblk13), cfblk71/1
  cfblk225/3(cfblk15) -> cfblk107/1, cfblk237/2(cfblk6)
  cfblk220/1(cfblk2) -> cfblk212/1(cfblk1)
  cfblk164/1 -> cfblk217/1(cfblk1)
  cfblk223/2(cfblk13) -> cfblk66/2
  cfblk223/3(cfblk14) -> cfblk106/1
  cfblk205/2(cfblk10) -> cfblk32/1
  cfblk46/1 -> cfblk92/1
  cfblk210/2(cfblk12) -> cfblk186/1
  cfblk84/1 -> cfblk216/3(cfblk11)
  cfblk246/4(cfblk14) -> cfblk25/1, cfblk249/2(cfblk12)
  cfblk52/1 -> cfblk93/1
  cfblk220/2(cfblk11) -> cfblk201/3(cfblk13)
  cfblk150/1 -> cfblk252/2(cfblk10)
  cfblk240/4(cfblk17) -> cfblk265/1, cfblk269/1, cfblk270/1
  cfblk250/2(cfblk15) -> cfblk119/1
  cfblk229/2(cfblk12) -> cfblk76/1
  cfblk229/3(cfblk13) -> cfblk125/1
  cfblk229/4(cfblk14) -> cfblk7/1
  cfblk204/3(cfblk13) -> cfblk96/1
  cfblk172/1 -> cfblk199/Action
  cfblk172/2 -> cfblk200/Action
  cfblk173/1 -> cfblk201/Action
  cfblk173/2 -> cfblk202/Action
  cfblk174/1 -> cfblk203/Action
  cfblk174/2 -> cfblk204/Action
  cfblk175/1 -> cfblk205/Action
  cfblk175/2 -> cfblk206/Action
  cfblk176/1 -> cfblk207/Action
  cfblk176/2 -> cfblk208/Action
  cfblk177/1 -> cfblk209/Action
  cfblk177/2 -> cfblk210/Action
  cfblk178/1 -> cfblk211/Action
  cfblk178/2 -> cfblk212/Action
  cfblk179/1 -> cfblk213/Action
  cfblk179/2 -> cfblk214/Action
  cfblk180/1 -> cfblk215/Action
  cfblk180/2 -> cfblk216/Action
  cfblk181/1 -> cfblk217/Action
  cfblk181/2 -> cfblk218/Action
  cfblk182/1 -> cfblk219/Action
  cfblk182/2 -> cfblk220/Action
  cfblk183/1 -> cfblk221/Action
  cfblk183/2 -> cfblk222/Action
  cfblk184/1 -> cfblk223/Action
  cfblk184/2 -> cfblk224/Action
  cfblk185/1 -> cfblk225/Action
  cfblk185/2 -> cfblk226/Action
  cfblk186/1 -> cfblk227/Action
  cfblk186/2 -> cfblk228/Action
  cfblk187/1 -> cfblk229/Action
  cfblk187/2 -> cfblk230/Action
  cfblk188/1 -> cfblk231/Action
  cfblk188/2 -> cfblk232/Action
  cfblk189/1 -> cfblk233/Action
  cfblk189/2 -> cfblk234/Action
  cfblk190/1 -> cfblk235/Action
  cfblk190/2 -> cfblk236/Action
  cfblk191/1 -> cfblk237/Action
  cfblk191/2 -> cfblk238/Action
  cfblk192/1 -> cfblk239/Action
  cfblk192/2 -> cfblk240/Action
  cfblk193/1 -> cfblk241/Action
  cfblk193/2 -> cfblk242/Action
  cfblk194/1 -> cfblk243/Action
  cfblk194/2 -> cfblk244/Action
  cfblk195/1 -> cfblk245/Action
  cfblk195/2 -> cfblk246/Action
  cfblk196/1 -> cfblk247/Action
  cfblk196/2 -> cfblk248/Action
  cfblk197/1 -> cfblk249/Action
  cfblk197/2 -> cfblk250/Action
  cfblk198/1 -> cfblk251/Action
  cfblk198/2 -> cfblk252/Action
  cfblk253/1 -> cfblk219/2(cfblk10)
  cfblk254/1 -> cfblk220/3(cfblk10)
  cfblk212/2(cfblk16) -> cfblk255/1
  cfblk255/1 -> cfblk252/1(cfblk1)
  cfblk252/1(cfblk2) -> cfblk256/1
  cfblk256/1 -> cfblk214/1(cfblk1)
  cfblk257/1 -> cfblk218/3(cfblk14)
  cfblk258/1 -> cfblk208/1(cfblk1)
  cfblk208/2(cfblk13) -> cfblk259/1
  cfblk259/1 -> cfblk207/2(cfblk13)
  cfblk199/1(cfblk2) -> cfblk260/1
  cfblk260/1 -> cfblk245/1(cfblk1)
  cfblk199/2(cfblk7) -> cfblk261/1
  cfblk261/1 -> cfblk215/3(cfblk14)
  cfblk199/3(cfblk8) -> cfblk262/1
  cfblk262/1 -> cfblk241/1(cfblk1)
  cfblk240/2(cfblk15) -> cfblk263/1
  cfblk263/1 -> cfblk189/1
  cfblk240/3(cfblk16) -> cfblk264/1
  cfblk264/1 -> cfblk220/1(cfblk1)
  cfblk265/1 -> cfblk248/2(cfblk8)
  cfblk266/1 -> cfblk251/2(cfblk8)
  cfblk56/1 -> cfblk267/1
  cfblk267/1 -> cfblk1/1
  cfblk228/1(cfblk2) -> cfblk268/1
  cfblk268/1 -> cfblk215/1(cfblk1)
  cfblk269/1 -> cfblk218/2(cfblk13)
  cfblk270/1 -> cfblk210/4(cfblk11)
  cfblk224/2(cfblk12) -> cfblk271/1
  cfblk271/1 -> cfblk198/1
  cfblk272/1 -> cfblk184/1
  cfblk273/1 -> cfblk220/2(cfblk9)
  cfblk274/1 -> cfblk212/2(cfblk15)
  cfblk275/1 -> cfblk216/4(cfblk12)
  cfblk23/1 -> cfblk276/1
  cfblk276/1 -> cfblk213/1(cfblk1)
  cfblk277/1 -> cfblk48/2
  cfblk57/1 -> cfblk278/1
  cfblk278/1 -> cfblk242/1(cfblk1)
  cfblk279/1 -> cfblk238/4(cfblk8)
  cfblk221/1(cfblk2) -> cfblk280/1
  cfblk280/1 -> cfblk216/1(cfblk1)
  cfblk250/1(cfblk2) -> cfblk281/1
  cfblk281/1 -> cfblk247/1(cfblk1)
  cfblk44/1 -> cfblk282/1
  cfblk282/1 -> cfblk246/1(cfblk1)
  cfblk246/1(cfblk2) -> cfblk283/1
  cfblk283/1 -> cfblk215/2(cfblk13)
  cfblk231/1(cfblk2) -> cfblk284/1
  cfblk284/1 -> cfblk210/1(cfblk1)
  cfblk231/2(cfblk15) -> cfblk285/1
  cfblk285/1 -> cfblk216/2(cfblk10)
  cfblk241/2(cfblk10) -> cfblk286/1
  cfblk286/1 -> cfblk209/2(cfblk8)
  cfblk287/1 -> cfblk210/3(cfblk10)
  cfblk34/1 -> cfblk288/1
  cfblk288/1 -> cfblk187/1
  cfblk204/2(cfblk12) -> cfblk289/1
  cfblk289/1 -> cfblk214/3(cfblk13)
  cfblk290/1 -> cfblk87/1
  cfblk59/1 -> cfblk291/1
  cfblk291/1 -> cfblk223/1(cfblk1)
  cfblk218/3(cfblk16) -> cfblk292/1
  cfblk292/1 -> cfblk59/1
  cfblk293/1 -> cfblk214/4(cfblk14), cfblk88/1, cfblk11/1
  cfblk209/1(cfblk2) -> cfblk294/1
  cfblk294/1 -> cfblk78/1

== system crash_original/cfblk163 ==
  Demux : Demux  Tag=STV Demux  Outputs=1
      settings: DisplayOption=none
  FromWs : FromWorkspace  Tag=STV FromWs  VariableName=tuvar
      SigBuilderData=|
      | common.afterFinalStr = 'Extrapolate'
      | common.sampleTime = 0
      | dataSet.timeRange = [0 10]
      | dataSet.name = 'Group 1'
      | sbobj.Groups.Name = 'Group 1'
      | sbobj.Groups.Signals.Name = 'Signal 1'
      | sbobj.Groups.Signals.XData = [0 4 4 6 6 10]
      | sbobj.Groups.Signals.YData = [0 0 1 1 0 0]
  Signal 1 : Outport  Tag=STV Outport  VectorParamsAs1DForOutWhenUnconnected=off
  wires:
  Demux/1 -> Signal 1/1
  FromWs/1 -> Demux/1

== system crash_original/cfblk167 ==
  Demux : Demux  Tag=STV Demux  Outputs=1
      settings: DisplayOption=none
  FromWs : FromWorkspace  Tag=STV FromWs  VariableName=tuvar
      SigBuilderData=|
      | common.afterFinalStr = 'Extrapolate'
      | common.sampleTime = 0
      | dataSet.timeRange = [0 10]
      | dataSet.name = 'Group 1'
      | sbobj.Groups.Name = 'Group 1'
      | sbobj.Groups.Signals.Name = 'Signal 1'
      | sbobj.Groups.Signals.XData = [0 4 4 6 6 10]
      | sbobj.Groups.Signals.YData = [0 0 1 1 0 0]
  Signal 1 : Outport  Tag=STV Outport  VectorParamsAs1DForOutWhenUnconnected=off
  wires:
  Demux/1 -> Signal 1/1
  FromWs/1 -> Demux/1

== system crash_original/cfblk199 ==
  cfblk1 : Inport
  Action Port : ActionPort  ActionPortLabel=if { }
  cfblk10 : DataTypeConversion
  cfblk11 : DataTypeConversion
  cfblk3 : UnitDelay  SampleTime=-1  HasFrameUpgradeWarning=on
  cfblk4 : DiscreteStateSpace  SampleTime=-1
  cfblk5 : slpidlib/PID Controller  Controller=PID  Form=Parallel  TimeDomain=Discrete-time  UseExternalTs=off  SampleTime=-1  IntegratorMethod=Forward Euler  FilterMethod=Forward Euler  ControllerParametersSource=internal  P=1  I=1  D=0  UseFilter=on  N=100  TunerSelectOption=Transfer Function Based (PID Tuner App)  InitialConditionSource=internal  InitialConditionForIntegrator=0  InitialConditionForFilter=0  DifferentiatorICPrevScaledInput=0  ExternalReset=none  TrackingMode=off  Kt=1  LimitOutput=off  SatLimitsSource=internal  UpperSaturationLimit=inf  LowerSaturationLimit=-inf  LinearizeAsGain=off  AntiWindupMode=none  Kb=1  POutMin=[]  POutMax=[]  IOutMin=[]  IOutMax=[]  DOutMin=[]  DOutMax=[]  NOutMin=[]  NOutMax=[]  SumOutMin=[]  SumOutMax=[]  SaturationOutMin=[]  SaturationOutMax=[]  PParamMin=[]  PParamMax=[]  IParamMin=[]  IParamMax=[]  DParamMin=[]  DParamMax=[]  NParamMin=[]  NParamMax=[]  KbParamMin=[]  KbParamMax=[]  KtParamMin=[]  KtParamMax=[]  KbOutMin=[]  KbOutMax=[]  KtOutMin=[]  KtOutMax=[]  IntegratorOutMin=[]  IntegratorOutMax=[]  FilterOutMin=[]  FilterOutMax=[]  SumI1OutMin=[]  SumI1OutMax=[]  SumI2OutMin=[]  SumI2OutMax=[]  SumI3OutMin=[]  SumI3OutMax=[]  SumI4OutMin=[]  SumI4OutMax=[]  SumDOutMin=[]  SumDOutMax=[]  DifferentiatorOutMin=[]  DifferentiatorOutMax=[]  FilterDiffOutCoefMin=[]  FilterDiffOutCoefMax=[]  ReciprocalOutMin=[]  ReciprocalOutMax=[]  SumDenOutMin=[]  SumDenOutMax=[]  SumNumOutMin=[]  SumNumOutMax=[]  DivideOutMin=[]  DivideOutMax=[]  UdiffTsProdOutMin=[]  UdiffTsProdOutMax=[]  NTsProdOutMin=[]  NTsProdOutMax=[]  UintegralTsProdOutMin=[]  UintegralTsProdOutMax=[]  UngainTsProdOutMin=[]  UngainTsProdOutMax=[]  IntegratorContinuousStateAttributes=''  IntegratorStateMustResolveToSignalObject=off  IntegratorRTWStateStorageClass=Auto  FilterContinuousStateAttributes=''  FilterStateMustResolveToSignalObject=off  FilterRTWStateStorageClass=Auto  ParallelPVariant=InternalParameters  IdealPVariant=Disabled  IVariant=InternalParameters  DVariant=InternalParameters  IntegratorVariant=Discrete  SatVariant=Disabled  AWVariant=Passthrough  PCopyVariant=Disabled  TRVariant=Disabled  FdbkBlocksVariant=Forward  IdealPFdbkVariant=Disabled  SatFdbkVariant=Disabled  DerivativeFilterVariant=ForwardEulerFilter  NVariant=InternalParameters  NCopyVariant=Disabled  FilterICVariant=InternalICsFilter  IntegratorICVariant=InternalICs  ExternalResetVariant=Disabled  TRSumVariant=Passthrough  SumFdbkVariant=Disabled  SumVariant=Sum_PID  TsampFilterVariant=InternalTs  TsampNgainVariant=Passthrough  TsampIntegralVariant=Passthrough  ExternalSaturationOutDataTypeStr=Inherit: Same as second input
  cfblk6 : slpidlib/PID Controller  Controller=PID  Form=Parallel  TimeDomain=Discrete-time  UseExternalTs=off  SampleTime=-1  IntegratorMethod=Forward Euler  FilterMethod=Forward Euler  ControllerParametersSource=internal  P=1  I=1  D=0  UseFilter=on  N=100  TunerSelectOption=Transfer Function Based (PID Tuner App)  InitialConditionSource=internal  InitialConditionForIntegrator=0  InitialConditionForFilter=0  DifferentiatorICPrevScaledInput=0  ExternalReset=none  TrackingMode=off  Kt=1  LimitOutput=off  SatLimitsSource=internal  UpperSaturationLimit=inf  LowerSaturationLimit=-inf  LinearizeAsGain=off  AntiWindupMode=none  Kb=1  POutMin=[]  POutMax=[]  IOutMin=[]  IOutMax=[]  DOutMin=[]  DOutMax=[]  NOutMin=[]  NOutMax=[]  SumOutMin=[]  SumOutMax=[]  SaturationOutMin=[]  SaturationOutMax=[]  PParamMin=[]  PParamMax=[]  IParamMin=[]  IParamMax=[]  DParamMin=[]  DParamMax=[]  NParamMin=[]  NParamMax=[]  KbParamMin=[]  KbParamMax=[]  KtParamMin=[]  KtParamMax=[]  KbOutMin=[]  KbOutMax=[]  KtOutMin=[]  KtOutMax=[]  IntegratorOutMin=[]  IntegratorOutMax=[]  FilterOutMin=[]  FilterOutMax=[]  SumI1OutMin=[]  SumI1OutMax=[]  SumI2OutMin=[]  SumI2OutMax=[]  SumI3OutMin=[]  SumI3OutMax=[]  SumI4OutMin=[]  SumI4OutMax=[]  SumDOutMin=[]  SumDOutMax=[]  DifferentiatorOutMin=[]  DifferentiatorOutMax=[]  FilterDiffOutCoefMin=[]  FilterDiffOutCoefMax=[]  ReciprocalOutMin=[]  ReciprocalOutMax=[]  SumDenOutMin=[]  SumDenOutMax=[]  SumNumOutMin=[]  SumNumOutMax=[]  DivideOutMin=[]  DivideOutMax=[]  UdiffTsProdOutMin=[]  UdiffTsProdOutMax=[]  NTsProdOutMin=[]  NTsProdOutMax=[]  UintegralTsProdOutMin=[]  UintegralTsProdOutMax=[]  UngainTsProdOutMin=[]  UngainTsProdOutMax=[]  IntegratorContinuousStateAttributes=''  IntegratorStateMustResolveToSignalObject=off  IntegratorRTWStateStorageClass=Auto  FilterContinuousStateAttributes=''  FilterStateMustResolveToSignalObject=off  FilterRTWStateStorageClass=Auto  ParallelPVariant=InternalParameters  IdealPVariant=Disabled  IVariant=InternalParameters  DVariant=InternalParameters  IntegratorVariant=Discrete  SatVariant=Disabled  AWVariant=Passthrough  PCopyVariant=Disabled  TRVariant=Disabled  FdbkBlocksVariant=Forward  IdealPFdbkVariant=Disabled  SatFdbkVariant=Disabled  DerivativeFilterVariant=ForwardEulerFilter  NVariant=InternalParameters  NCopyVariant=Disabled  FilterICVariant=InternalICsFilter  IntegratorICVariant=InternalICs  ExternalResetVariant=Disabled  TRSumVariant=Passthrough  SumFdbkVariant=Disabled  SumVariant=Sum_PID  TsampFilterVariant=InternalTs  TsampNgainVariant=Passthrough  TsampIntegralVariant=Passthrough  ExternalSaturationOutDataTypeStr=Inherit: Same as second input
  cfblk9 : Delay
  cfblk2 : Outport  VectorParamsAs1DForOutWhenUnconnected=off
  cfblk7 : Outport  Port=2  VectorParamsAs1DForOutWhenUnconnected=off
  cfblk8 : Outport  Port=3  VectorParamsAs1DForOutWhenUnconnected=off
  wires:
  cfblk1/1 -> cfblk3/1
  cfblk3/1 -> cfblk7/1, cfblk2/1
  cfblk4/1 -> cfblk6/1, cfblk11/1
  cfblk6/1 -> cfblk9/1
  cfblk9/1 -> cfblk4/1
  cfblk5/1 -> cfblk10/1
  cfblk10/1 -> cfblk8/1
  cfblk11/1 -> cfblk5/1

== system crash_original/cfblk200 ==
  cfblk1 : Inport
  cfblk8 : Inport  Port=2
  Action Port : ActionPort  ActionPortLabel=else { }
  cfblk3 : UnitDelay  SampleTime=-1  HasFrameUpgradeWarning=on
  cfblk4 : DiscreteTransferFcn
  cfblk5 : DiscreteStateSpace  SampleTime=-1
  cfblk6 : Delay  ShowEnablePort=on
      settings: InputPortMap=u0,e6
  cfblk7 : simulink/Discrete/Transfer Fcn First Order  PoleZ=0.95  ICPrevOutput=0.0  DoSatur=off
  cfblk9 : Delay
  cfblk2 : Outport  VectorParamsAs1DForOutWhenUnconnected=off
  wires:
  cfblk7/1 -> cfblk2/1
  cfblk8/1 -> cfblk4/1
  cfblk1/1 -> cfblk7/1
  cfblk3/1 -> cfblk6/1
  cfblk5/1 -> cfblk6/2
  cfblk4/1 -> cfblk5/1
  cfblk6/1 -> cfblk9/1
  cfblk9/1 -> cfblk3/1
